simulink model "s11_18"  (Simulink 6.6)
settings: Solver=ode45  StartTime=0.0  StopTime=T  MaxStep=0.01  RelTol=1e-3
values from neighbouring files (symbols this model uses):
  T_s = 0.01    [i11_18.m]
  theta_0 = -pi/2    (= -1.57079632679)    [i11_18.m]
  x_0 = -1    [i11_18.m]
  y_0 = -2    [i11_18.m]
undefined symbols (not defined in the file or in its folder): post_reg, wrap
settings Model: Creator=marilena  LastModifiedBy=giuseppe  ExtModeAutoUpdateStatusClock=off
settings OptimizationCC: InitFltsAndDblsToZero=off
settings HardwareCC: TargetHWDeviceType=32-bit Generic

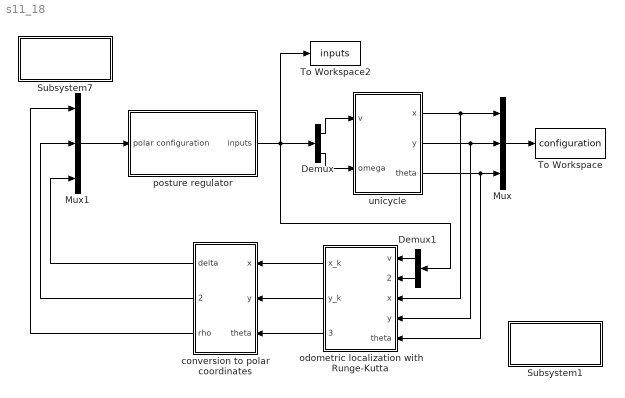
== system s11_18 ==
  Demux : Demux  Outputs=2
  Demux1 : Demux  Orientation=left  Outputs=2
  Mux : Mux  Inputs=3
  Mux1 : Mux  Inputs=3
  Subsystem1 : Subsystem
      settings: OpenFcn=p11_18
      mask Display: disp('plot')
  Subsystem7 : Subsystem
      settings: OpenFcn=i11_18
      mask Display: disp('variables \n initialization')
  To Workspace : ToWorkspace  VariableName=configuration  SaveFormat=Structure With Time
  To Workspace2 : ToWorkspace  VariableName=inputs  SaveFormat=Structure With Time
  conversion to polar coordinates : Subsystem  Orientation=left
  odometric localization with Runge-Kutta : Subsystem  Orientation=left
  posture regulator : Subsystem
  unicycle : Subsystem
  wires:
  Mux/1 -> To Workspace/1
  unicycle/3(theta) -> Mux/3, odometric localization with Runge-Kutta/5(theta)
  unicycle/1(x) -> Mux/1, odometric localization with Runge-Kutta/3(x)
  Mux1/1 -> posture regulator/1(polar configuration)
  posture regulator/1(inputs) -> Demux/1, To Workspace2/1, Demux1/1
  unicycle/2(y) -> Mux/2, odometric localization with Runge-Kutta/4(y)
  Demux/1 -> unicycle/1(v)
  Demux/2 -> unicycle/2(omega)
  Demux1/1 -> odometric localization with Runge-Kutta/1(v)
  Demux1/2 -> odometric localization with Runge-Kutta/2(omega)
  odometric localization with Runge-Kutta/1(x_k) -> conversion to polar coordinates/1(x)
  odometric localization with Runge-Kutta/2(y_k) -> conversion to polar coordinates/2(y)
  odometric localization with Runge-Kutta/3(theta_k) -> conversion to polar coordinates/3(theta)
  conversion to polar coordinates/1(delta) -> Mux1/3
  conversion to polar coordinates/2(gamma) -> Mux1/2
  conversion to polar coordinates/3(rho) -> Mux1/1

== system s11_18/Subsystem1 ==

== system s11_18/Subsystem7 ==

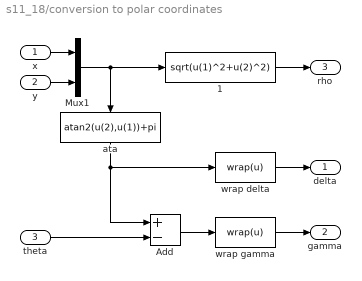
== system s11_18/conversion to polar coordinates ==
  x : Inport  OutDataType=fixdt(1,16,0)  OutScaling=[]
  y : Inport  Port=2  OutDataType=fixdt(1,16,0)  OutScaling=[]
  theta : Inport  Port=3  OutDataType=fixdt(1,16,0)  OutScaling=[]
  " 1" : Fcn  Expr=sqrt(u(1)^2+u(2)^2)
  Add : Sum  Inputs=+-  OutScaling=2^-10
  Mux1 : Mux  Inputs=2
  ata : Fcn  Orientation=down  Expr=atan2(u(2),u(1))+pi
  wrap delta : MATLABFcn  MATLABFcn=wrap(u)
  wrap gamma : MATLABFcn  MATLABFcn=wrap(u)
  delta : Outport  OutDataType=fixdt(1,16,0)  OutScaling=[]
  gamma : Outport  Port=2  OutDataType=fixdt(1,16,0)  OutScaling=[]
  rho : Outport  Port=3  OutDataType=fixdt(1,16,0)  OutScaling=[]
  wires:
  Mux1/1 -> " 1"/1, ata/1
  ata/1 -> Add/1, wrap delta/1
  x/1 -> Mux1/1
  " 1"/1 -> rho/1
  y/1 -> Mux1/2
  theta/1 -> Add/2
  wrap delta/1 -> delta/1
  Add/1 -> wrap gamma/1
  wrap gamma/1 -> gamma/1

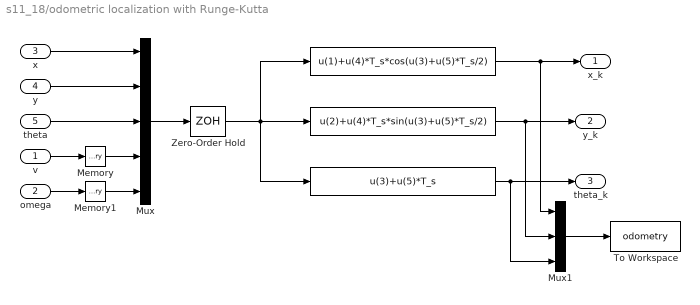
== system s11_18/odometric localization with Runge-Kutta ==
  v : Inport  OutDataType=fixdt(1,16,0)  OutScaling=[]
  omega : Inport  Port=2  OutDataType=fixdt(1,16,0)  OutScaling=[]
  x : Inport  Port=3  OutDataType=fixdt(1,16,0)  OutScaling=[]
  y : Inport  Port=4  OutDataType=fixdt(1,16,0)  OutScaling=[]
  theta : Inport  Port=5  OutDataType=fixdt(1,16,0)  OutScaling=[]
  " " : Fcn  Expr=u(1)+u(4)*T_s*cos(u(3)+u(5)*T_s/2)
  "  " : Fcn  Expr=u(2)+u(4)*T_s*sin(u(3)+u(5)*T_s/2)
  "   " : Fcn  Expr=u(3)+u(5)*T_s
  Memory : Memory
  Memory1 : Memory
  Mux : Mux  Inputs=5
  Mux1 : Mux  Inputs=3
  To Workspace : ToWorkspace  VariableName=odometry  SaveFormat=Structure With Time
  Zero-Order Hold : ZeroOrderHold  SampleTime=T_s
  x_k : Outport  OutDataType=fixdt(1,16,0)  OutScaling=[]
  y_k : Outport  Port=2  OutDataType=fixdt(1,16,0)  OutScaling=[]
  theta_k : Outport  Port=3  OutDataType=fixdt(1,16,0)  OutScaling=[]
  wires:
  Mux/1 -> Zero-Order Hold/1
  " "/1 -> x_k/1, Mux1/1
  x/1 -> Mux/1
  y/1 -> Mux/2
  "  "/1 -> y_k/1, Mux1/2
  "   "/1 -> theta_k/1, Mux1/3
  Zero-Order Hold/1 -> "  "/1, " "/1, "   "/1
  v/1 -> Memory/1
  omega/1 -> Memory1/1
  Memory/1 -> Mux/4
  Memory1/1 -> Mux/5
  theta/1 -> Mux/3
  Mux1/1 -> To Workspace/1

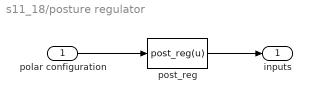
== system s11_18/posture regulator ==
  polar configuration : Inport
  post_reg : MATLABFcn  Tag={'prova'}  Description=cartesian regulator  MATLABFcn=post_reg(u)  Output1D=off
  inputs : Outport
  wires:
  polar configuration/1 -> post_reg/1
  post_reg/1 -> inputs/1

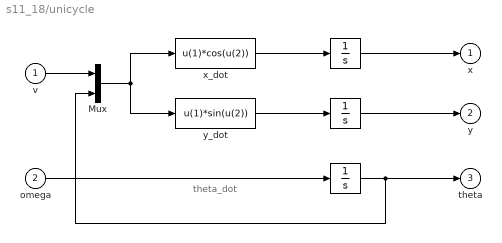
== system s11_18/unicycle ==
  note: theta_dot
  v : Inport  OutDataType=fixdt(1,16,0)  OutScaling=[]
  omega : Inport  Port=2  OutDataType=fixdt(1,16,0)  OutScaling=[]
  " " : Integrator  InitialCondition=theta_0
  "   " : Integrator  InitialCondition=x_0
  "    " : Integrator  InitialCondition=y_0
  Mux : Mux  Inputs=2
  x_dot : Fcn  Expr=u(1)*cos(u(2))
  y_dot : Fcn  Expr=u(1)*sin(u(2))
  x : Outport  OutDataType=fixdt(1,16,0)  OutScaling=[]
  y : Outport  Port=2  OutDataType=fixdt(1,16,0)  OutScaling=[]
  theta : Outport  Port=3  OutDataType=fixdt(1,16,0)  OutScaling=[]
  wires:
  v/1 -> Mux/1
  omega/1 -> " "/1
  x_dot/1 -> "   "/1
  y_dot/1 -> "    "/1
  " "/1 -> Mux/2, theta/1
  Mux/1 -> x_dot/1, y_dot/1
  "   "/1 -> x/1
  "    "/1 -> y/1
